simulink model "P1_Ex3"  (R2018a)
settings: Solver=FixedStepAuto  StartTime=0.0  StopTime=15  RelTol=1e-3
undefined symbols (not defined in the file): Kp, Tg, Ts, Vmax, Vmin
libraries: arduinolib x2
settings Model: SimulationMode=external  ExtModeTrigDuration=2  Creator=Eneko Lerma  LastModifiedBy=Eneko Lerma
settings OptimizationCC: EnhancedBackFolding=on  PassReuseOutputArgsAs=Individual arguments  MaxStackSize=64  OptimizeBlockOrder=speed  DifferentSizesBufferReuse=on  OptimizationCustomize=off
settings DebuggingCC: ParameterPrecisionLossMsg=none  ParameterTunabilityLossMsg=error
settings HardwareCC: ProdBitPerPointer=32  ProdBitPerSizeT=32  ProdBitPerPtrDiffT=32  ProdLargestAtomicInteger=Long  ProdLargestAtomicFloat=Double  ProdWordSize=32  ProdHWDeviceType=ARM Compatible->ARM Cortex
settings SFSimCC: MATLABDynamicMemAlloc=off
settings RTWCC: SystemTargetFile=ert.tlc  HardwareBoard=Arduino Due  TLCOptions=-aInlineSetEventsForThisBaseRateFcn=TLC_FALSE -aSuppressMultiTaskScheduler=TLC_FALSE -aRateBasedStepFcn=1  TemplateMakefile=ert_default_tmf  GenerateReport=on  Toolchain=Arduino ARM  BuildConfiguration=Faster Runs  IncludeHyperlinkInReport=on  LaunchReport=on  GenerateTraceInfo=on  GenerateTraceReport=on  GenerateTraceReportSl=on  GenerateTraceReportSf=on  GenerateTraceReportEml=on
settings CodeAppCC: ForceParamTrailComments=on  IgnoreCustomStorageClasses=off  OperatorAnnotations=on  SimulinkDataObjDesc=on  SFDataObjDesc=on  InsertBlockDesc=on
settings ERTTargetCC: SupportContinuousTime=on  SupportVariableSizeSignals=on

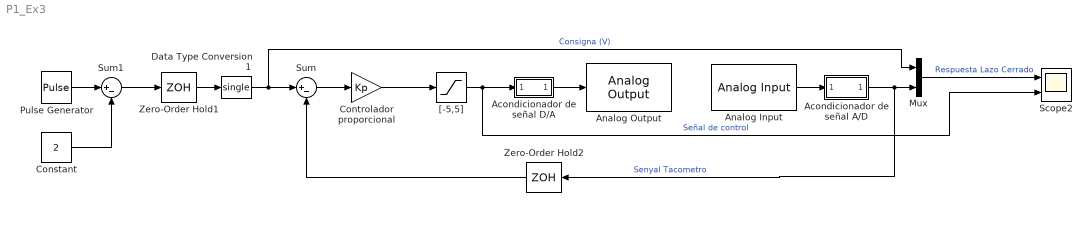
== system P1_Ex3 ==
  Acondicionador de señal A/D : Subsystem
  Acondicionador de señal D/A : Subsystem
  Analog Input : arduinolib/Analog Input  pinNumber=2  ReadResultsOnly=off  ConversionTriggerSource=Software  ExternalTriggerType=uint32(0)  OutputDataType=uint16  EnableConversionCompleteNotify=off  EnableOuputStatus=off  SampleTime=Tg  blockPlatform=arduino
  Analog Output : arduinolib/Analog Output  DACpin=DAC1  blockPlatform=arduino
      settings: SourceProductName=Simulink Support Package for Arduino Hardware  SourceProductBaseCode=ARDUINO
  Constant : Constant  Value=2  SampleTime=Ts
  Controlador proporcional : Gain  Gain=Kp
  Data Type Conversion1 : DataTypeConversion  OutDataTypeStr=single
  Mux : Mux  Inputs=2
  Pulse Generator : DiscretePulseGenerator  PulseType=Time based  Amplitude=4  Period=5  PulseWidth=50  SampleTime=Ts
  Scope2 : Scope  NumInputPorts=2
  Sum : Sum  Inputs=|+-
  Sum1 : Sum  Inputs=|+-
  Zero-Order Hold1 : ZeroOrderHold  SampleTime=Ts
  Zero-Order Hold2 : ZeroOrderHold  SampleTime=Ts
  "[-5,5]" : Saturate  UpperLimit=Vmax  LowerLimit=Vmin  OutDataTypeStr=single
  wires:
  Mux/1 -> Scope2/1  "Respuesta Lazo Cerrado"
  "[-5,5]"/1 -> Acondicionador de señal D/A/1("  "), Scope2/2  "Señal de control"
  Acondicionador de señal D/A/1(" ") -> Analog Output/1
  Sum1/1 -> Zero-Order Hold1/1
  Analog Input/1 -> Acondicionador de señal A/D/1(" ")
  Acondicionador de señal A/D/1(" ") -> Zero-Order Hold2/1, Mux/2  "Senyal Tacometro"
  Data Type Conversion1/1 -> Sum/1, Mux/1  "Consigna (V)"
  Sum/1 -> Controlador proporcional/1
  Controlador proporcional/1 -> "[-5,5]"/1
  Pulse Generator/1 -> Sum1/1
  Constant/1 -> Sum1/2
  Zero-Order Hold2/1 -> Sum/2
  Zero-Order Hold1/1 -> Data Type Conversion1/1

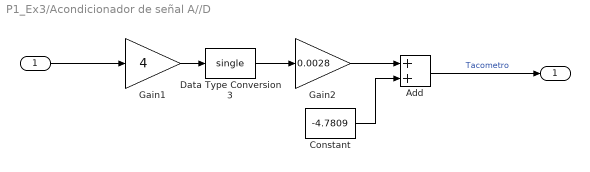
== system P1_Ex3/Acondicionador de señal A//D ==
  " " : Inport
  Add : Sum  AccumDataTypeStr=single
  Constant : Constant  Value=-4.7809  OutDataTypeStr=single  SampleTime=Ts
  Data Type Conversion3 : DataTypeConversion  OutDataTypeStr=single
  Gain1 : Gain  Gain=4  OutDataTypeStr=uint16
  Gain2 : Gain  Gain=0.0028  OutDataTypeStr=single
  " " : Outport
  wires:
  Gain1/1 -> Data Type Conversion3/1
  " "/1 -> Gain1/1
  Add/1 -> " "/1  "Tacometro"
  Gain2/1 -> Add/1
  Constant/1 -> Add/2
  Data Type Conversion3/1 -> Gain2/1

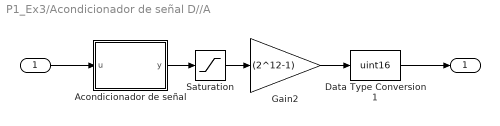
== system P1_Ex3/Acondicionador de señal D//A ==
  "  " : Inport  OutDataTypeStr=single
  Acondicionador de señal : MATLAB Function  TreatAsAtomicUnit=on
  Data Type Conversion1 : DataTypeConversion  OutDataTypeStr=uint16
  Gain2 : Gain  Gain=(2^12-1)  OutDataTypeStr=single
  Saturation : Saturate  UpperLimit=1  LowerLimit=0  OutDataTypeStr=single
  " " : Outport  OutDataTypeStr=uint16
  wires:
  Saturation/1 -> Gain2/1
  Data Type Conversion1/1 -> " "/1
  Acondicionador de señal/1(y) -> Saturation/1
  "  "/1 -> Acondicionador de señal/1(u)
  Gain2/1 -> Data Type Conversion1/1

== matlab function P1_Ex3/Acondicionador de señal D//A/Acondicionador de señal ==
  data: u input; y output
function y = fcn(u)
y =0.1342*u+0.3926;
